simulink model "Eg11_1"  (R2018a)
settings: Solver=VariableStepAuto  StartTime=0.0  StopTime=10.0  RelTol=1e-3
settings Model: Creator=wangluo  LastModifiedBy=wangluo

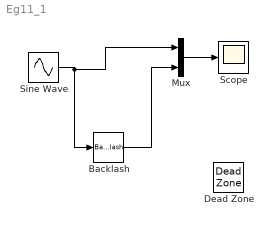
== system Eg11_1 ==
  Backlash : Backlash
  Dead Zone : DeadZone  SaturateOnIntegerOverflow=on
  Mux : Mux  Inputs=2
  Scope : Scope
  Sine Wave : Sin  SampleTime=0
  wires:
  Sine Wave/1 -> Backlash/1, Mux/1
  Mux/1 -> Scope/1
  Backlash/1 -> Mux/2
